simulink model "slbb"  (Simulink 7.5)
settings: Solver=ode5  SolverMode=SingleTasking  StartTime=0.0  StopTime=1000  FixedStep=0.1  MaxStep=0.1  RelTol=1e-3  AbsTol=1e-6
PreLoadFcn:
  | initbb
undefined symbols (not defined in the file or in its folder): init_cond
libraries: fuzblock x1
CloseFcn:
  | AnimBbFigTitle = [winName, ': Ball & Beam Animation']; AnimBbFigH = findobj(0,'Name',AnimBbFigTitle); close(AnimBbFigH)
settings Model: Creator=pascal  LastModifiedBy=rchen
settings DataIOCC: LimitDataPoints=off  SaveOutput=off  SaveTime=off
settings OptimizationCC: BlockReduction=off  BooleanDataType=off  InitFltsAndDblsToZero=on
settings DebuggingCC: SaveWithParameterizedLinksMsg=none  SignalResolutionControl=TryResolveAllWithWarning  SolverPrmCheckMsg=none  MultiTaskDSMMsg=warning  MultiTaskCondExecSysMsg=none  StrictBusMsg=None
settings HardwareCC: TargetUnknown=on
settings RTWCC: TemplateMakefile=grt_unix.tmf  IncludeERTFirstTime=on
settings GRTTargetCC: TargetFcnLib=ansi_tfl_tmw.mat

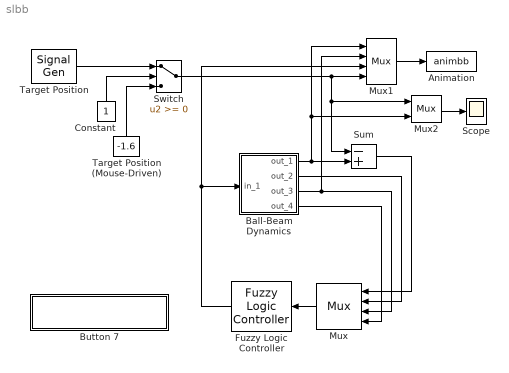
== system slbb ==
  Animation : S-Function  FunctionName=animbb  EnableBusSupport=off
  Ball-Beam Dynamics : Subsystem  mask(Ball-Beam Dynamics){init_cond =[0 0 0 0]}
      mask prompts: init_cond  "Initial Conditions:"
      mask help: Ball-Beam Dynamics
      mask Help: Dynamics of the ball and beam system
      mask Display: plot(-4,-1,4,5,[0 -1 1 0 3 2.9 -3 -2.9 0],[2 0 0 2 3 3.1 1.1 1.0 2],0.3*cos(linspace(0,2*pi,9))+2,0.3*sin(linspace(0,2*pi,9))+3.1);
  Button 7 : Subsystem
      settings: OpenFcn=initbb
      mask Display: disp('Variable Initialization')
  Constant : Constant  OutDataType=sfix(16)  OutScaling=2^0
  Fuzzy Logic Controller : fuzblock/Fuzzy Logic  Controller  SystemSampleTime=-1  fis=fismatrix
  Mux : Mux
  Mux1 : Mux
  Mux2 : Mux  Inputs=2
  Scope : Scope
      settings: TickLabels=on  TimeRange=10.000000  YMin=-2  YMax=2  DataFormat=Array
  Sum : Sum  Inputs=-+  OutDataType=sfix(16)  OutScaling=2^0  SaturateOnIntegerOverflow=on  InputSameDT=on  OutDataTypeStr=Inherit: Same as first input
  Switch : Switch  SaturateOnIntegerOverflow=on  InputSameDT=on
  Target Position : SignalGenerator  WaveForm=square  Amplitude=1.600000  Frequency=0.500000  Units=rad/sec
  Target Position (Mouse-Driven) : Constant  Value=-1.6  OutDataType=sfix(16)  OutScaling=2^0
  wires:
  Mux2/1 -> Scope/1
  Switch/1 -> Mux2/1, Sum/1, Mux1/4
  Sum/1 -> Mux/1
  Ball-Beam Dynamics/2(out_2) -> Mux/2
  Ball-Beam Dynamics/3(out_3) -> Mux/3, Mux1/2
  Ball-Beam Dynamics/4(out_4) -> Mux/4
  Target Position (Mouse-Driven)/1 -> Switch/3
  Constant/1 -> Switch/2
  Target Position/1 -> Switch/1
  Ball-Beam Dynamics/1(out_1) -> Mux2/2, Mux1/1, Sum/2
  Mux/1 -> Fuzzy Logic Controller/1
  Mux1/1 -> Animation/1
  Fuzzy Logic Controller/1 -> Mux1/3, Ball-Beam Dynamics/1(in_1)

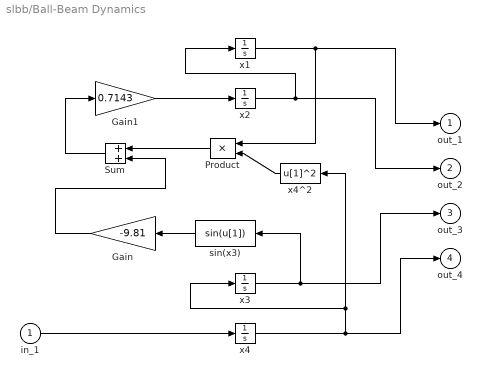
== system slbb/Ball-Beam Dynamics ==
  in_1 : Inport  OutDataType=sfix(16)  OutScaling=2^0
  Gain : Gain  Gain=-9.81  ParameterDataType=sfix(16)  ParameterScaling=2^0  OutDataType=sfix(16)  OutScaling=2^0  SaturateOnIntegerOverflow=on  OutDataTypeStr=Inherit: Same as input  ParamDataTypeStr=Inherit: Same as input
  Gain1 : Gain  Gain=0.7143  ParameterDataType=sfix(16)  ParameterScaling=2^0  OutDataType=sfix(16)  OutScaling=2^0  SaturateOnIntegerOverflow=on  OutDataTypeStr=Inherit: Same as input  ParamDataTypeStr=Inherit: Same as input
  Product : Product  OutDataType=sfix(16)  OutScaling=2^0  SaturateOnIntegerOverflow=on  RndMeth=Zero  InputSameDT=on  OutDataTypeStr=Inherit: Same as first input
  Sum : Sum  OutDataType=sfix(16)  OutScaling=2^0  SaturateOnIntegerOverflow=on  InputSameDT=on  OutDataTypeStr=Inherit: Same as first input
  sin(x3) : Fcn
  x1 : Integrator  InitialCondition=init_cond(1)
  x2 : Integrator  InitialCondition=init_cond(2)
  x3 : Integrator  InitialCondition=init_cond(3)
  x4 : Integrator  InitialCondition=init_cond(4)
  x4^2 : Fcn  Expr=u[1]^2
  out_1 : Outport  OutDataType=sfix(16)  OutScaling=2^0  InitialOutput=0
  out_2 : Outport  Port=2  OutDataType=sfix(16)  OutScaling=2^0  InitialOutput=0
  out_3 : Outport  Port=3  OutDataType=sfix(16)  OutScaling=2^0  InitialOutput=0
  out_4 : Outport  Port=4  OutDataType=sfix(16)  OutScaling=2^0  InitialOutput=0
  wires:
  in_1/1 -> x4/1
  x2/1 -> out_2/1, x1/1
  x1/1 -> Product/1, out_1/1
  x4^2/1 -> Product/2
  sin(x3)/1 -> Gain/1
  Product/1 -> Sum/1
  Gain/1 -> Sum/2
  Sum/1 -> Gain1/1
  Gain1/1 -> x2/1
  x4/1 -> x3/1, x4^2/1, out_4/1
  x3/1 -> sin(x3)/1, out_3/1

== system slbb/Button 7 ==
